simulink model "w2_prob3_214869"  (R2020a)
settings: Solver=ode45  StartTime=0.0  StopTime=120  RelTol=1e-3
undefined symbols (not defined in the file or in its folder): b, m
settings Model: DataDictionary=sonali.sldd  Creator=sonal  LastModifiedBy=sonal

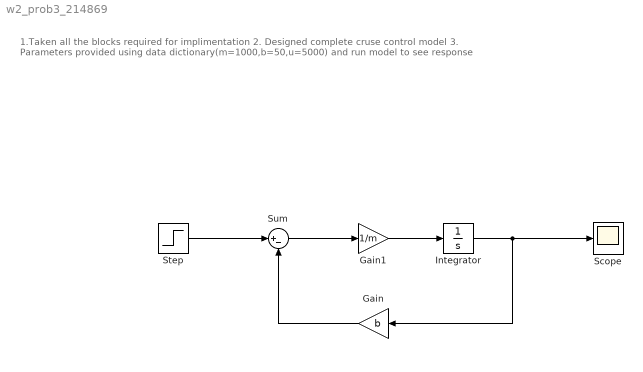
== system w2_prob3_214869 ==
  note: 1.Taken all the blocks required for implimentation
      | 2. Designed complete cruse control model
      | 3. Parameters provided using data dictionary(m=1000,b=50,u=5000)
      | and run model to see response
  Gain : Gain  Gain=b
  Gain1 : Gain  Gain=1/m
  Integrator : Integrator
  Scope : Scope
  Step : Step  Time=0  After=u  SampleTime=0
  Sum : Sum  Inputs=|+-
  wires:
  Step/1 -> Sum/1
  Sum/1 -> Gain1/1
  Gain1/1 -> Integrator/1
  Integrator/1 -> Scope/1, Gain/1
  Gain/1 -> Sum/2
